simulink model "td2simAM"  (Simulink 7.5)
settings: Solver=ode45  StartTime=0.0  StopTime=Tsim  RelTol=1e-3
values from neighbouring files (symbols this model uses):
  nu_m = 10    [td3filtre.m]
undefined symbols (not defined in the file or in its folder): A, B
settings Model: Creator=gscorlet  LastModifiedBy=gscorlet
settings DataIOCC: Refine=10
settings OptimizationCC: InitFltsAndDblsToZero=on
settings DebuggingCC: SaveWithParameterizedLinksMsg=none  SignalResolutionControl=TryResolveAllWithWarning  MultiTaskDSMMsg=warning  MultiTaskCondExecSysMsg=none  StrictBusMsg=Warning
settings RTWCC: IncludeERTFirstTime=on
settings GRTTargetCC: TargetFcnLib=ansi_tfl_tmw.mat

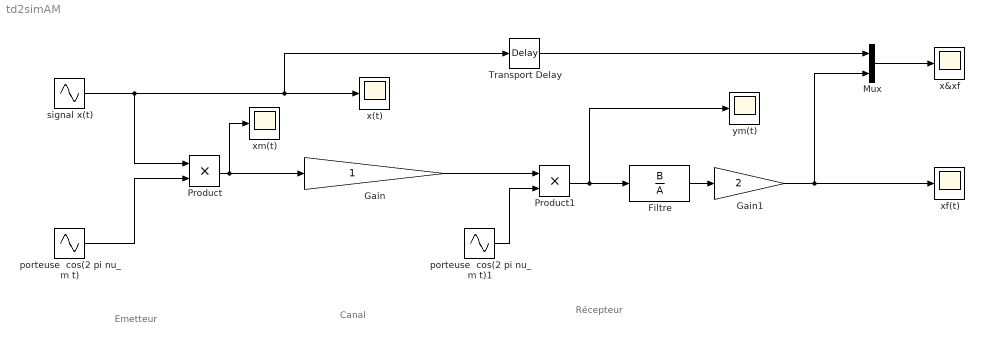
== system td2simAM ==
  note: Emetteur
  note: Canal
  note: Récepteur
  Filtre : TransferFcn  Numerator=B  Denominator=A
  Gain : Gain  ParameterDataType=sfix(16)  ParameterScaling=2^0  OutDataType=sfix(16)  OutScaling=2^0
  Gain1 : Gain  Gain=2  ParameterDataType=sfix(16)  ParameterScaling=2^0  OutDataType=sfix(16)  OutScaling=2^0
  Mux : Mux  Inputs=2
  Product : Product  OutDataType=sfix(16)  OutScaling=2^0  RndMeth=Zero
  Product1 : Product  OutDataType=sfix(16)  OutScaling=2^0  RndMeth=Zero
  Transport Delay : TransportDelay  DelayTime=0
  porteuse  cos(2 pi nu_m t) : Sin  Amplitude=1  Bias=0  Frequency=2*pi*nu_m  Phase=0  Samples=10  SampleTime=0  Offset=0
  porteuse  cos(2 pi nu_m t)1 : Sin  Amplitude=1  Bias=0  Frequency=2*pi*nu_m  Phase=0  Samples=10  SampleTime=0  Offset=0
  signal x(t) : Sin  Amplitude=1  Bias=0  Frequency=2*pi*1  Phase=pi/2  Samples=10  SampleTime=0  Offset=0
  x&xf : Scope
      settings: SaveName=ScopeData4
  x(t) : Scope
      settings: SaveName=ScopeData2
  xf(t) : Scope
      settings: SaveName=ScopeData3
  xm(t) : Scope
  ym(t) : Scope
  wires:
  porteuse  cos(2 pi nu_m t)/1 -> Product/2
  Product/1 -> Gain/1, xm(t)/1
  Gain/1 -> Product1/1
  Product1/1 -> ym(t)/1, Filtre/1
  Filtre/1 -> Gain1/1
  porteuse  cos(2 pi nu_m t)1/1 -> Product1/2
  Mux/1 -> x&xf/1
  Gain1/1 -> xf(t)/1, Mux/2
  Transport Delay/1 -> Mux/1
  signal x(t)/1 -> Transport Delay/1, x(t)/1, Product/1
